simulink model "goingbackup"  (Simulink 7.5)
settings: Solver=ode3  StartTime=0.0  StopTime=inf  FixedStep=.05  RelTol=1e-3
undefined symbols (not defined in the file or in its folder): CR, serial
libraries: instrumentlib x3, simulink x2, realtime_pacer_lib x1
settings Model: Creator=TCA  LastModifiedBy=meuser
settings OptimizationCC: InitFltsAndDblsToZero=on
settings DebuggingCC: StrictBusMsg=Warning

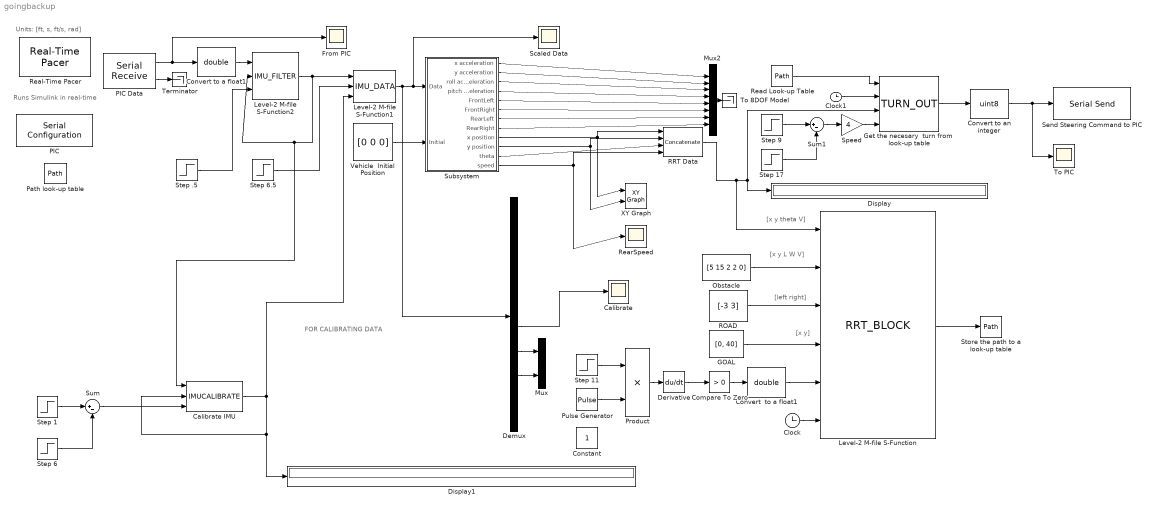
== system goingbackup ==
  note: [x y theta V]
  note: [x y L W V]
  note: [left right]
  note: [x y]
  note: Runs Simulink
      |  in real-time
  note: Units: [ft, s, ft/s, rad]
  note: FOR CALIBRATING DATA
  Calibrate : Scope
      settings: TimeRange=8  YMin=-1  YMax=1  SaveName=ScopeData3
  Calibrate IMU : M-S-Function  FunctionName=IMUCALIBRATE  Parameters=3
  Clock : Clock
      settings: Decimation=10
  Clock1 : Clock
      settings: Decimation=10
  Compare To Zero : simulink/Logic and Bit Operations/Compare To Zero  SystemSampleTime=-1  relop=>  LogicOutDataTypeMode=uint8  ZeroCross=off
  Constant : Constant  OutDataType=fixdt(1, 16)  OutScaling=2^0
  Convert to a float1 : DataTypeConversion  OutDataTypeMode=double  OutDataTypeStr=double  SaturateOnIntegerOverflow=on  RndMeth=Zero
  Convert  to a float1 : DataTypeConversion  OutDataTypeMode=double  OutDataTypeStr=double  SaturateOnIntegerOverflow=on  RndMeth=Zero
  Convert to an integer : DataTypeConversion  OutDataTypeMode=uint8  OutDataTypeStr=uint8  SampleTime=.05  SaturateOnIntegerOverflow=on  RndMeth=Zero
  Demux : Demux  Outputs=10
  Derivative : Derivative
  Display : Display
  Display1 : Display
  From PIC : Scope
      settings: TimeRange=10  YMin=0  YMax=225
  GOAL : Constant  Value=[0, 40]  VectorParams1D=off
  Get the necesary  turn from  look-up table : M-S-Function  FunctionName=TURN_OUT  Parameters=4
  Level-2 M-file S-Function : M-S-Function  FunctionName=RRT_BLOCK  Parameters=6
  Level-2 M-file S-Function1 : M-S-Function  FunctionName=IMU_DATA  Parameters=3
  Level-2 M-file S-Function2 : M-S-Function  FunctionName=IMU_FILTER  Parameters=3
  Mux : Mux  Inputs=2
  Mux2 : Mux  Inputs=8
  Obstacle : Constant  Value=[5 15 2 2 0]  VectorParams1D=off
  PIC : instrumentlib/Serial Configuration  Priority=-200000  DialogController=instrumentcreatedialog  DialogControllerArgs=DataTag0  ComPortMenu=COM5  ComPort=COM5  ObjConstructor=serial('COM5');  BaudRate=115200  DataBits=8  Parity=none  StopBits=1  FlowControl=none  Timeout=10  ByteOrder=LittleEndian
  PIC Data : instrumentlib/Serial Receive  DialogController=instrumentcreatedialog  DialogControllerArgs=DataTag1  ComPortMenu=COM5  ComPort=COM5  ObjConstructor=serial('COM5');  Terminator=CR ('\r')  DataSize="[1  16]"  DataType=uint8  EnableBlockingMode=off  ActionDataUnavailable=Output last received value  CustomValue=0  SampleTime=.05
  Path look-up table : DataStoreMemory  DataStoreName=Path  ReadBeforeWriteMsg=warning  WriteAfterWriteMsg=warning  WriteAfterReadMsg=warning  InitialValue=zeros(50, 6)  VectorParams1D=off
  Product : Product  OutDataType=fixdt(1, 16)  OutScaling=2^0  RndMeth=Zero
  Pulse Generator : DiscretePulseGenerator  PulseType=Time based  Amplitude=1  Period=1  PulseWidth=50  PhaseDelay=0  SampleTime=1
  ROAD : Constant  Value=[-3 3]  VectorParams1D=off
  RRT Data : Concatenate  NumInputs=4  Mode=Multidimensional array  ConcatenateDimension=2
  Read Look-up Table : DataStoreRead  DataStoreName=Path  SampleTime=0
  Real-Time Pacer : realtime_pacer_lib/Real-Time Pacer  simTimePerRealTime=1
  RearSpeed : Scope
      settings: TimeRange=8  YMin=-1  YMax=1  SaveName=ScopeData2
  Scaled Data : Scope
      settings: TimeRange=10  YMin=-2  YMax=2.5
  Send Steering Command to PIC : instrumentlib/Serial Send  DialogController=instrumentcreatedialog  DialogControllerArgs=DataTag2  ComPortMenu=COM5  ComPort=COM5  ObjConstructor=serial('COM5');  Header=250  Terminator=<none>  EnableBlockingMode=off
  Speed : Gain  Gain=4  ParameterDataType=fixdt(1, 16)  ParameterScaling=2^0  OutDataType=fixdt(1, 16)  OutScaling=2^0
  Step .5 : Step  Time=.5  SampleTime=0
  Step 1 : Step  SampleTime=0
  Step 11 : Step  Time=11  SampleTime=0
  Step 17 : Step  Time=17  SampleTime=0
  Step 6 : Step  Time=6  SampleTime=0
  Step 6.5 : Step  Time=6.5  SampleTime=0
  Step 9 : Step  Time=9  SampleTime=0
  Store the path to a look-up table : DataStoreWrite  DataStoreName=Path  SampleTime=-1
  Subsystem : Subsystem
  Sum : Sum  Inputs=|+-  OutDataType=fixdt(1, 16)  OutScaling=2^0
  Sum1 : Sum  Inputs=|+-  OutDataType=fixdt(1, 16)  OutScaling=2^0
  Terminator : Terminator
  To 8DOF Model : Terminator
  To PIC : Scope
      settings: TimeRange=10  YMin=120  YMax=250  SaveName=ScopeData4
  Vehicle  Initial Position : Constant  Value=[0 0 0]  VectorParams1D=off
  XY Graph : simulink/Sinks/XY Graph  SystemSampleTime=-1  xmin=-4  xmax=4  ymin=-1  ymax=25  st=-1
  wires:
  ROAD/1 -> Level-2 M-file S-Function/3
  GOAL/1 -> Level-2 M-file S-Function/4
  Compare To Zero/1 -> Convert  to a float1/1
  Level-2 M-file S-Function/1 -> Store the path to a look-up table/1
  Convert  to a float1/1 -> Level-2 M-file S-Function/5
  Derivative/1 -> Compare To Zero/1
  Clock/1 -> Level-2 M-file S-Function/6
  Clock1/1 -> Get the necesary  turn from  look-up table/2
  Convert to an integer/1 -> Send Steering Command to PIC/1, To PIC/1
  PIC Data/1 -> Convert to a float1/1, From PIC/1
  Obstacle/1 -> Level-2 M-file S-Function/2
  PIC Data/2 -> Terminator/1
  Level-2 M-file S-Function1/1 -> Subsystem/1(Data), Scaled Data/1, Demux/1
  Subsystem/9(x position) -> RRT Data/1, XY Graph/1
  Subsystem/10(y position) -> RRT Data/2, XY Graph/2
  Subsystem/11(theta) -> RRT Data/3
  Subsystem/12(speed) -> RRT Data/4, RearSpeed/1
  RRT Data/1 -> Level-2 M-file S-Function/1, Get the necesary  turn from  look-up table/3, Display/1
  Step .5/1 -> Level-2 M-file S-Function2/3
  Vehicle  Initial Position/1 -> Subsystem/2(Initial)
  Read Look-up Table/1 -> Get the necesary  turn from  look-up table/1
  Speed/1 -> Get the necesary  turn from  look-up table/4
  Convert to a float1/1 -> Level-2 M-file S-Function2/1
  Level-2 M-file S-Function2/1 -> Level-2 M-file S-Function1/1, Calibrate IMU/1, Level-2 M-file S-Function2/2
  Subsystem/1(x acceleration) -> Mux2/1
  Subsystem/2(y acceleration) -> Mux2/2
  Subsystem/3(roll acceleration) -> Mux2/3
  Subsystem/4(pitch acceleration) -> Mux2/4
  Mux2/1 -> To 8DOF Model/1
  Calibrate IMU/1 -> Display1/1, Calibrate IMU/2, Level-2 M-file S-Function1/3
  Step 1/1 -> Sum/1
  Step 6/1 -> Sum/2
  Sum/1 -> Calibrate IMU/3
  Step 6.5/1 -> Level-2 M-file S-Function1/2
  Step 9/1 -> Sum1/1
  Step 17/1 -> Sum1/2
  Sum1/1 -> Speed/1
  Demux/7 -> Mux/1
  Demux/8 -> Mux/2
  Step 11/1 -> Product/1
  Product/1 -> Derivative/1
  Demux/6 -> Calibrate/1
  Subsystem/8(RearRight) -> Mux2/8
  Subsystem/7(RearLeft) -> Mux2/7
  Subsystem/6(FrontRight) -> Mux2/6
  Subsystem/5(FrontLeft) -> Mux2/5
  Pulse Generator/1 -> Product/2
  Get the necesary  turn from  look-up table/1 -> Convert to an integer/1

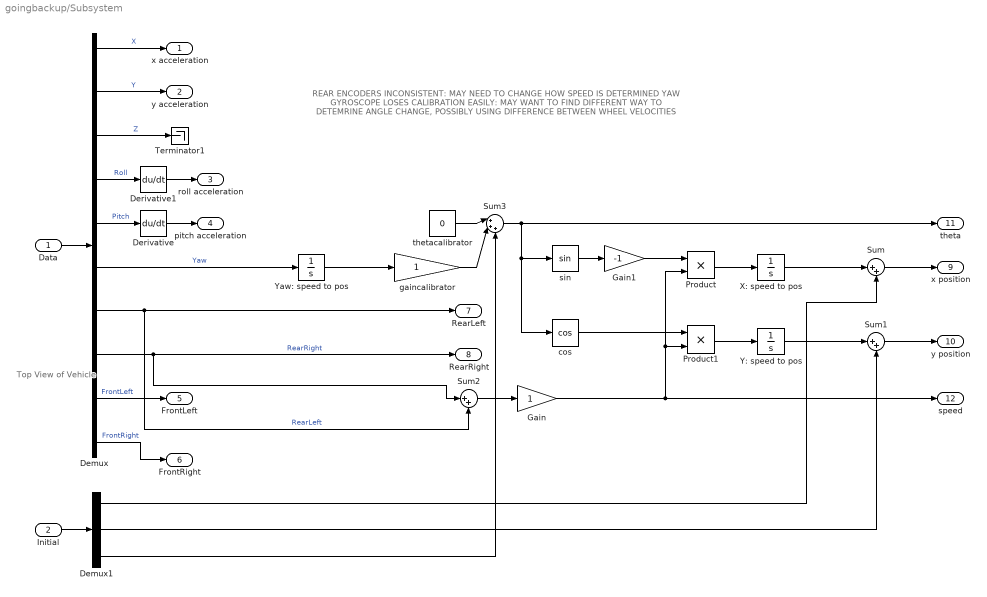
== system goingbackup/Subsystem ==
  note: Top View
      | of Vehicle
  note: REAR ENCODERS INCONSISTENT: MAY NEED TO CHANGE HOW SPEED IS DETERMINED
      | YAW GYROSCOPE LOSES CALIBRATION EASILY: MAY WANT TO FIND DIFFERENT WAY TO DETEMRINE
      | ANGLE CHANGE, POSSIBLY USING DIFFERENCE BETWEEN WHEEL VELOCITIES
  Data : Inport
  Initial : Inport  Port=2  OutDataType=fixdt(1, 16)  OutScaling=2^0
  Demux : Demux  Outputs=10
  Demux1 : Demux  Outputs=3
  Derivative : Derivative
  Derivative1 : Derivative
  Gain : Gain  ParameterDataType=fixdt(1, 16)  ParameterScaling=2^0  OutDataType=fixdt(1, 16)  OutScaling=2^0
  Gain1 : Gain  Gain=-1  ParameterDataType=fixdt(1, 16)  ParameterScaling=2^0  OutDataType=fixdt(1, 16)  OutScaling=2^0
  Product : Product  OutDataType=fixdt(1, 16)  OutScaling=2^0  RndMeth=Zero
  Product1 : Product  OutDataType=fixdt(1, 16)  OutScaling=2^0  RndMeth=Zero
  Sum : Sum  Inputs=|++  OutDataType=fixdt(1, 16)  OutScaling=2^0
  Sum1 : Sum  Inputs=|++  OutDataType=fixdt(1, 16)  OutScaling=2^0
  Sum2 : Sum  Inputs=|++  OutDataType=fixdt(1, 16)  OutScaling=2^0
  Sum3 : Sum  Inputs=|+++  OutDataType=fixdt(1, 16)  OutScaling=2^0
  Terminator1 : Terminator
  X: speed to pos : Integrator
  Y: speed to pos : Integrator
  Yaw: speed to pos : Integrator
  cos : Trigonometry  Operator=cos
  gaincalibrator : Gain  ParameterDataType=fixdt(1, 16)  ParameterScaling=2^0  OutDataType=fixdt(1, 16)  OutScaling=2^0
  sin : Trigonometry
  thetacalibrator : Constant  Value=0  OutDataType=fixdt(1, 16)  OutScaling=2^0
  x acceleration : Outport
  y acceleration : Outport  Port=2
  roll acceleration : Outport  Port=3
  pitch acceleration : Outport  Port=4
  FrontLeft : Outport  Port=5
  FrontRight : Outport  Port=6
  RearLeft : Outport  Port=7
  RearRight : Outport  Port=8
  x position : Outport  Port=9
  y position : Outport  Port=10
  theta : Outport  Port=11
  speed : Outport  Port=12
  wires:
  Demux/1 -> x acceleration/1  "X"
  Demux/2 -> y acceleration/1  "Y"
  Demux/3 -> Terminator1/1  "Z"
  Demux/6 -> Yaw: speed to pos/1  "Yaw"
  Sum1/1 -> y position/1
  Data/1 -> Demux/1
  Sum3/1 -> theta/1, sin/1, cos/1
  Demux/7 -> RearLeft/1, Sum2/2  "RearLeft"
  Demux/8 -> RearRight/1, Sum2/1  "RearRight"
  Demux/9 -> FrontLeft/1  "FrontLeft"
  Demux/10 -> FrontRight/1  "FrontRight"
  Sum2/1 -> Gain/1
  Sum/1 -> x position/1
  sin/1 -> Gain1/1
  thetacalibrator/1 -> Sum3/1
  Gain1/1 -> Product/1
  cos/1 -> Product1/1
  Product1/1 -> Y: speed to pos/1
  Product/1 -> X: speed to pos/1
  X: speed to pos/1 -> Sum/1
  Y: speed to pos/1 -> Sum1/1
  Gain/1 -> speed/1, Product1/2, Product/2
  Derivative/1 -> pitch acceleration/1
  Derivative1/1 -> roll acceleration/1
  Demux/4 -> Derivative1/1  "Roll"
  Demux/5 -> Derivative/1  "Pitch"
  Yaw: speed to pos/1 -> gaincalibrator/1
  gaincalibrator/1 -> Sum3/2
  Initial/1 -> Demux1/1
  Demux1/1 -> Sum/2
  Demux1/2 -> Sum1/2
  Demux1/3 -> Sum3/3
